simulink model "Ejercicio4_simulink"  (R2016a)
settings: Solver=VariableStepAuto  StartTime=0.0  StopTime=800  RelTol=1e-3
settings Model: Creator=estebanza  LastModifiedBy=estebanza

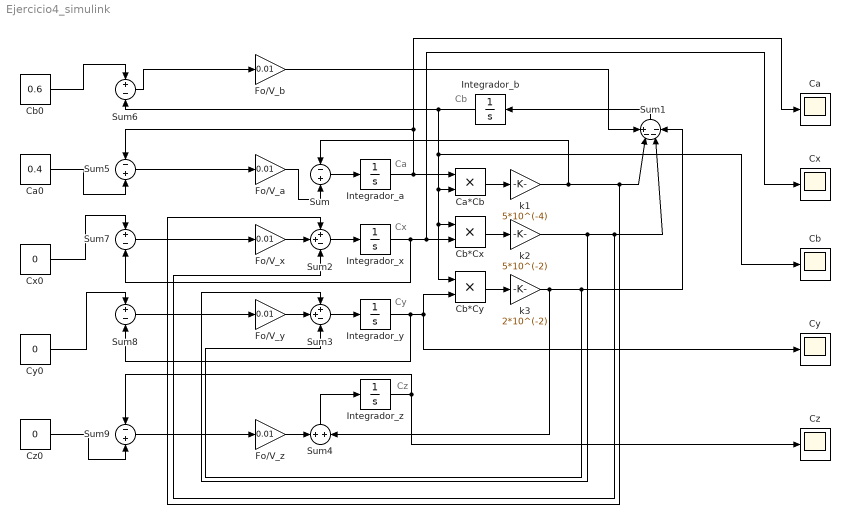
== system Ejercicio4_simulink ==
  note: Cx
  note: Cb
  note: Ca
  note: Cy
  note: Cz
  Ca : Scope
  Ca*Cb : Product
  Ca0 : Constant  Value=0.4
  Cb : Scope
  Cb*Cx : Product
  Cb*Cy : Product
  Cb0 : Constant  Value=0.6
  Cx : Scope
  Cx0 : Constant  Value=0
  Cy : Scope
  Cy0 : Constant  Value=0
  Cz : Scope
  "Cz0 " : Constant  Value=0
  Fo/V_a : Gain  Gain=0.01
  Fo/V_b : Gain  Gain=0.01
  Fo/V_x : Gain  Gain=0.01
  Fo/V_y : Gain  Gain=0.01
  Fo/V_z : Gain  Gain=0.01
  Integrador_a : Integrator
  Integrador_b : Integrator
  Integrador_x : Integrator
  Integrador_y : Integrator
  Integrador_z : Integrator
  Sum : Sum  Inputs=-+
  Sum1 : Sum  Inputs=+---
  Sum2 : Sum  Inputs=++-
  Sum3 : Sum  Inputs=++-
  Sum4 : Sum
  Sum5 : Sum  Inputs=-+
  Sum6 : Sum  Inputs=+-
  Sum7 : Sum  Inputs=+-
  Sum8 : Sum  Inputs=+-
  Sum9 : Sum  Inputs=-+
  k1 : Gain  Gain=5*10^(-4)
  k2 : Gain  Gain=5*10^(-2)
  k3 : Gain  Gain=2*10^(-2)
  wires:
  Sum/1 -> Integrador_a/1
  k1/1 -> Sum2/1, Sum1/2, Sum/1
  k2/1 -> Sum2/3, Sum1/3, Sum3/1
  k3/1 -> Sum4/2, Sum1/4, Sum3/3
  Sum1/1 -> Integrador_b/1
  Cb*Cx/1 -> k2/1
  Cb*Cy/1 -> k3/1
  Integrador_x/1 -> Cb*Cx/2, Cx/1, Sum7/2
  Sum2/1 -> Integrador_x/1
  Ca*Cb/1 -> k1/1
  Fo/V_b/1 -> Sum1/1
  Fo/V_x/1 -> Sum2/2
  Integrador_y/1 -> Cb*Cy/2, Cy/1, Sum8/2
  Sum3/1 -> Integrador_y/1
  Sum4/1 -> Integrador_z/1
  Cb0/1 -> Sum6/1
  Cx0/1 -> Sum7/1
  Cy0/1 -> Sum8/1
  "Cz0 "/1 -> Sum9/2
  Integrador_z/1 -> Cz/1, Sum9/1
  Sum9/1 -> Fo/V_z/1
  Fo/V_z/1 -> Sum4/1
  Sum5/1 -> Fo/V_a/1
  Fo/V_a/1 -> Sum/2
  Ca0/1 -> Sum5/2
  Integrador_a/1 -> Sum5/1, Ca/1, Ca*Cb/1
  Integrador_b/1 -> Cb*Cy/1, Cb*Cx/1, Ca*Cb/2, Cb/1, Sum6/2
  Sum6/1 -> Fo/V_b/1
  Sum7/1 -> Fo/V_x/1
  Fo/V_y/1 -> Sum3/2
  Sum8/1 -> Fo/V_y/1
